simulink model "CM620A_MotAg0Meas"  (R2013b)
settings: Solver=FixedStepDiscrete  SolverMode=SingleTasking  StartTime=0.0  StopTime=1  FixedStep=0.0000625  RelTol=1e-3
undefined symbols (not defined in the file): ARCHGLBPRM_2PI_ULS_F32, COEFFTBLELMSIZE_CNT_U08, COEFFTBLSIZE_CNT_U08, CORRNTBLAGSTEPSIZE_MATRAD_F32, CORRNTBLSIDXOFFS_CNT_U16, CORRNTBLSIZE_CNT_U16, CORRNTBLSIZEMASK_CNT_U08, FLTINJ_MOTAG0MEAS_MOTCTRLMOTAG0MECL, FLTINJ_MOTAG0MEAS_TESTOK, MotAg0PrtclFlt, MOTAG0PRTCLFLTFAILSTEP_CNT_U16, MOTAG0PRTCLFLTPASSSTEP_CNT_U16, MOTAGDELTAPERCORRNPT_CNT_U16, MOTAGIDXMASK_CNT_U16, MotCtrlMotAg0ErrReg, NtcSts1, sigbuilder_block, SNSRAGMASK_CNT_U32, SNSRERRMASK_CNT_U32, SNSRERRNTCMASK_CNT_U08, SNSRVLTGFLTMASK_CNT_U32, SPIPARMASK_CNT_U32
libraries: simulink x28, FloatToFixd x1, NxtrMax x1, NxtrLim x1
(part 1 of 4)
settings Model: RequirementInfo="{}  %GIDa_ca294f38_ed7c_4fb9_8c54_f4d56271bfc7"  ModifiedHistory=Rev 008: Updated model to Matlab 2013B, added comments to show requirement linkage  Creator=nz3zln  LastModifiedBy=TZBSJD
settings SolverCC: AutoInsertRateTranBlk=on  InsertRTBMode=Always
settings DataIOCC: LimitDataPoints=off  SaveFormat=Structure  ReturnWorkspaceOutputs=on
settings OptimizationCC: BlockReduction=off  InlineParams=on  ZeroExternalMemoryAtStartup=off  ZeroInternalMemoryAtStartup=off  OptimizeModelRefInitCode=on  LifeSpan=1
settings DebuggingCC: SignalInfNanChecking=error  SignalRangeChecking=warning  UnderspecifiedInitializationDetection=Simplified  SolverPrmCheckMsg=error  InheritedTsInSrcMsg=error  DiscreteInheritContinuousMsg=error  SingleTaskRateTransMsg=error  TasksWithSamePriorityMsg=error  SigSpecEnsureSampleTimeMsg=error  CheckMatrixSingularityMsg=error  ParameterUnderflowMsg=error  ParameterPrecisionLossMsg=error  ParameterTunabilityLossMsg=error  FixptConstUnderflowMsg=warning  FixptConstOverflowMsg=warning  VectorMatrixConversionMsg=error  SignalLabelMismatchMsg=error  UnconnectedInputMsg=error  UnconnectedOutputMsg=error  UnconnectedLineMsg=error  SFcnCompatibilityMsg=error  UniqueDataStoreMsg=warning  BusObjectLabelMismatch=error  RootOutportRequireBusObject=error  AssertControl=DisableAll  ModelReferenceIOMsg=error  ModelReferenceVersionMismatchMessage=warning  ModelReferenceIOMismatchMessage=error  ModelReferenceCSMismatchMessage=warning  ModelReferenceDataLoggingMessage=error  StateNameClashWarn=warning  StrictBusMsg=ErrorOnBusTreatedAsVector  NonBusSignalsTreatedAsBus=error  SFUnexpectedBacktrackingDiag=error  SFInvalidInputDataAccessInChartInitDiag=error  SFNoUnconditionalDefaultTransitionDiag=error  SFTransitionOutsideNaturalParentDiag=error  SFUnconditionalTransitionShadowingDiag=error  SFUndirectedBroadcastEventsDiag=error
settings ModelReferenceCC: ModelReferenceNumInstancesAllowed=Single
settings RTWCC: SystemTargetFile=autosar.tlc  GenCodeOnly=on  TemplateMakefile=ert_default_tmf  Description=AUTOSAR  GenerateReport=on  ProcessScript=autosar_make_rtw_hook  LaunchReport=on
settings CodeAppCC: GenerateComments=off  IgnoreCustomStorageClasses=off  CustomSymbolStrType=$N$R$M  CustomSymbolStrBlkIO=$N$M  SimulinkBlockComments=off
settings STFCustomTargetCC: ParMdlRefBuildCompliant=on  CompOptLevelCompliant=on  IncludeMdlTerminateFcn=off  CombineOutputUpdateFcns=on  SuppressErrorStatus=on  ERTFirstTimeCompliant=on  ERTCustomFileBanners=on  SupportNonFinite=off  SupportComplex=off  SupportContinuousTime=off  SupportNonInlinedSFcns=off  MATLABClassNameForMDSCustomization=Simulink.SoftwareTarget.ERTCustomization  AutosarCompliant=on  GRTInterface=off  SystemTargetFile=autosar.tlc
settings ERTTargetCC: CodeReplacementLibrary=ANSI_C  ConcurrentExecutionCompliant=off  IncludeMdlTerminateFcn=off  SuppressErrorStatus=on  SupportNonFinite=off  SupportComplex=off  ModelStepFunctionPrototypeControlCompliant=off  CPPClassGenCompliant=off  AutosarCompliant=on  InlinedParameterPlacement=NonHierarchical  ERTCustomFileTemplate=example_file_process.tlc  EnableUserReplacementTypes=on

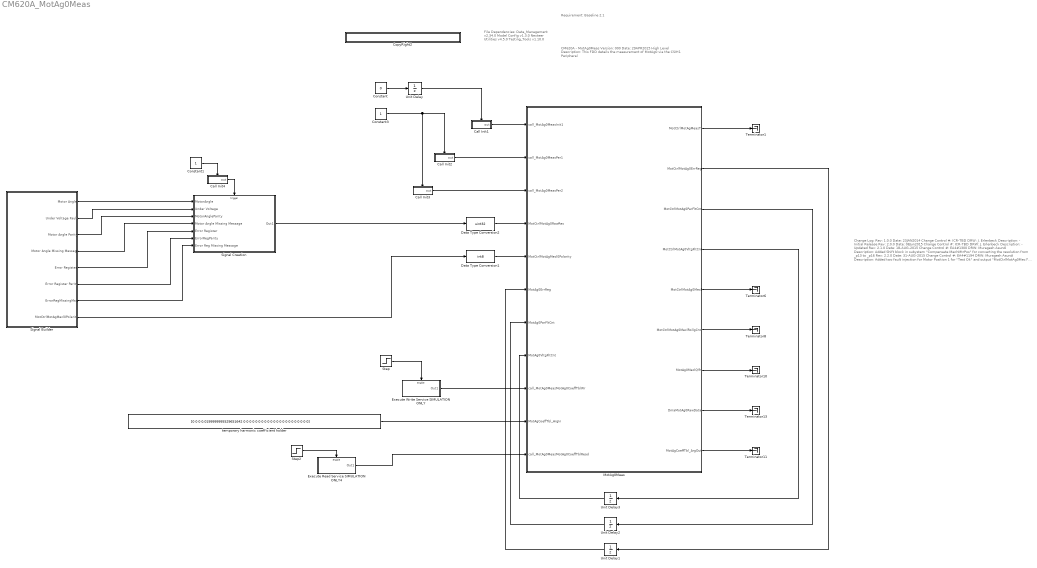
== system CM620A_MotAg0Meas ==
  note: CM620A - MotAg0Meas
      |
      | Version: 000
      | Date: 29APR2015
      |
      | High Level Description:
      | This FDD details the measurement of MotAg0 via the CSIH1 Peripheral
  note: Change Log:
      |
      | Rev: 1.0.0
      | Date: 23JAN2014
      | Change Control #: ICR-TBD
      | DRW: J. Erlenbeck
      | Description:
      | - Initial Release
      |
      | Rev: 2.0.0
      | Date: 08Jun2015
      | Change Control #: ICR-TBD
      | DRW: J. Erlenbeck
      | Description:
      | - Updated
      |
      | Rev: 2.1.0
      | Date: 18-AUG-2015
      | Change Control #: EA4#1300
      | DRW: Muragesh Asundi
      | Description: Added Shift block in subystem "Compensate MechMtrPos" for converting the resolution from _p13 to _p16
      |
      | Rev: 2.2.0
      | Date: 31-AUG-2015
      | Change Control #: EA4#1194
      | DRW: Muragesh Asundi
      | Description: Added two fault injection for Motor Position 1 for "Test Ok" and output "MotCtrlMotAg0Mecl"
      |
      | Rev: 2.3.0
      | Date: 09-SEP-2015
      | Change Control #: EA4#1404
      | DRW: J. Erlenbeck
      | Description: Updated for Anomaly fix to scaling
      |
      | Rev: 2.4.0
      | Date: 23-SEP-2015
      | Change Control #: EA4#1639
      | DRW: Muragesh Asundi
      | Description: Block "FltInj_u16" renamed to "FltInj_u0p16"
      |
      | Rev 3.0.0
      | Date - 30-Sep-2015
      | Change Control EA4#1725
      | DRW" Erlenbeck
      | Description: Changes to the Correction table process
      |
      | Rev 3.1.0
      | Date - 07-Oct-2015
      | Change Control EA4#1883
      | DRW" Erlenbeck
      | Description: Created routine in Init1 to initialize CSIH RAM to prevent ECC faults.  Place in some checks to to
      | verify denominator !=0 before division.
      |
      | Rev 3.2.0
      | Date - 18-Oct-2015
      | Change Control EA4#2085
      | DRW: Erlenbeck
      | Description: Removed routine in Init1 to initialize CSIH RAM to prevent ECC faults.  Changed some
      | typecasting in init function that prevented the function from running when NxtrMBDConfig.mat was run.
      | Replaced input signal creation from external file to one with signal builder.\
      |
      | Rev 3.2.1
      | Date - 18-Oct-2015
      | Change Control EA4#2085
      | DRW: Erlenbeck
      | Description: Minor changes needed for model to compile with NxtrMBDConfig.mat configuration.
      |
      | Rev 3.4.0
      | Date - 17-Dec-2015
      | Change Control EA4#3027
      | DRW: Erlenbeck
      | Description: Removed the read reset pointer.  Will be performed by the DMA.
      |
      | Rev 3.5.0
      | Date - 08-Mar-2016
      | Change Control EA4#3925, EA4#4645
      | DRW: Praveen(KPIT)
      | Description:
      | - M File change so that NVM MotAg0CoeffTbl.EngInit = []. Accordingly model updated to allign to this.
      | - As per anomaly CR EA4#3631, updated the variable MotCtrlMotAg0VltgFltCnt.WrittenIn field as MotAg1MeasPer1 in the .m file.
      |  -The maximum and minimum specified in the Data Type conversion block are removed and highlighted in the Model.
      |
      | Rev 3.6.0
      | Date - 07-Dec-2016
      | Change Control EA4#8812
      | DRW: Sai Desu
      | Description:
      | - Updated MotAg0VltgFltCnt.ReadIn in M-file from MotAg0MeasPer1 to MotAg0MeasPer2
  note: File Dependencies:
      | Data_Management v2.34.0
      | Model Config v1.3.0
      | Nexteer Utilities v4.5.0
      | Testing_Tools v1.10.0
  note: Requirement: Baseline 2.1
  Call Init1 : Subsystem  TreatAsAtomicUnit=on
  Call Init2 : Subsystem  TreatAsAtomicUnit=on
  Call Init3 : Subsystem  TreatAsAtomicUnit=on
  Call Init4 : Subsystem  TreatAsAtomicUnit=on
  Constant : Constant  Value=0  OutDataTypeStr=uint8
  Constant1 : Constant  OutDataTypeStr=int8
  Constant3 : Constant  OutDataTypeStr=int8
  CopyRight2 : Subsystem  Description=|  mask(Copyright Information){none=on}
      | Copyright info block.                                               
      |                                                                     
      | Place copyright information at the top of every subsystem in design.
      mask prompts: none "No parameters"
      mask help: Place copyright information at the top of every subsystem in design.
      mask Display:
      | NxtrConf = 'Nexteer Confidential';
      | 
      | sys = bdroot; %handle for the current model ("system")
      | first = get_param(sys,'Created');
      | first = first(end-3:end);  %year is last four digits
      | 
      | last = get_param(sys,'LastModifiedDate');
      | if isempty(last)
      |     last = datestr(now,'yyyy');
      | else
      |     last = last(end-3:end);
      | end
      | 
      | if strcmp(first,last)
      |     fprintf('%s -- Copyright %s Nexteer',NxtrConf,first)
      | else
      |     fprintf('%s -- %s%s- %s Nexteer',NxtrConf,char(169),first,last)
      | end
  Data Type Conversion1 : DataTypeConversion  OutDataTypeStr=int8
  Data Type Conversion2 : DataTypeConversion  OutDataTypeStr=uint32
  Execute Read Service SIMULATION ONLY4 : Subsystem  TreatAsAtomicUnit=on
  Execute Write Service SIMULATION ONLY : Subsystem  TreatAsAtomicUnit=on
  MotAg0Meas : Subsystem
  Signal Builder : Subsystem  Tag=STV Subsys  LoadFcn=sigbuilder_block('load');  StartFcn=sigbuilder_block('start');  StopFcn=sigbuilder_block('stop');  ClipboardFcn=sigbuilder_block('clipboard');  mask(Sigbuilder block){}
      mask help: Simulink:masks:SigbuilderBlock_MD
      mask init:
      | if ~strcmp(get_param(bdroot(gcbh),'SimulationStatus'),'stopped') tuvar = sigbuilder_block('maskInit'); end
      settings: CopyFcn=sigbuilder_block('copy');  DeleteFcn=sigbuilder_block('delete');  ModelCloseFcn=sigbuilder_block('modelClose');  PreSaveFcn=sigbuilder_block('preSave');  PauseFcn=sigbuilder_block('pause');  ContinueFcn=sigbuilder_block('continue');  NameChangeFcn=sigbuilder_block('namechange');  OpenFcn=sigbuilder_block('open',[306 215.379 548.69 396.621 ]);  CloseFcn=sigbuilder_block('close');
      mask Display: plot(0, 0, 100, 100,[2, 2, 32, 32, 2], [68, 8, 8, 68, 68],[32, 2], [38, 38], [32, 19, 2],[53, 60, 44], [32, 17, 17, 2],[16, 16, 31, 31]);txt = getActiveGroup(gcbh);text(2, 100, txt,'verticalAlignment', 'top');
  Signal Creation : Subsystem
  Step : Step  Time=0.05  SampleTime=0
  Step2 : Step  Time=0.8  SampleTime=0
  Terminator{1,6,8,10..11,13} (6 alike) : Terminator
  Unit Delay : UnitDelay  InitialCondition=1  SampleTime=-1
  Unit Delay1 : UnitDelay  SampleTime=-1
  Unit Delay2 : UnitDelay  SampleTime=-1
  Unit Delay3 : UnitDelay  SampleTime=-1
  temporary harmonic coefficient holder : Constant  Value=[0 0 0 0.0199999995529651642 0 0 0 0 0 0 0 0 0 0 0 0 0 0 0 0 0 0 0 0 0 0]  OutDataTypeStr=single
  wires:
  Constant/1 -> Unit Delay/1
  Unit Delay/1 -> Call Init1/Enable
  Constant3/1 -> Call Init2/Enable, Call Init3/Enable
  Call Init1/1(out) -> MotAg0Meas/1(call_MotAg0MeasInit1)
  Call Init2/1(out) -> MotAg0Meas/2(call_MotAg0MeasPer1)
  Signal Creation/1(Out1) -> Data Type Conversion2/1
  Data Type Conversion2/1 -> MotAg0Meas/4(MotCtrlMotAg0RawRes)
  Call Init3/1(out) -> MotAg0Meas/3(call_MotAg0MeasPer2)
  Step/1 -> Execute Write Service SIMULATION ONLY/Enable
  Execute Write Service SIMULATION ONLY/1(Out1) -> MotAg0Meas/9(call_MotAg0MeasMotAg0CoeffTblWr)
  MotAg0Meas/1(MotCtrlMotAgMeasTi) -> Terminator1/1
  MotAg0Meas/5(MotCtrlMotAg0Mecl) -> Terminator6/1
  MotAg0Meas/6(MotCtrlMotAg0MeclRollgCntr) -> Terminator8/1
  MotAg0Meas/7(MotAg0MeclQlfr) -> Terminator10/1
  MotAg0Meas/8(DmaMotAg0RawData) -> Terminator13/1
  Step2/1 -> Execute Read Service SIMULATION ONLY4/Enable
  Execute Read Service SIMULATION ONLY4/1(Out1) -> MotAg0Meas/11(call_MotAg0MeasMotAg0CoeffTblRead)
  temporary harmonic coefficient holder/1 -> MotAg0Meas/10(MotAgCoeffTbl_ArgIn)
  MotAg0Meas/9(MotAgCoeffTbl_ArgOut) -> Terminator11/1
  MotAg0Meas/2(MotCtrlMotAg0ErrReg) -> Unit Delay1/1
  Unit Delay1/1 -> MotAg0Meas/6(MotAg0ErrReg)
  MotAg0Meas/3(MotCtrlMotAg0ParFltCnt) -> Unit Delay2/1
  Unit Delay2/1 -> MotAg0Meas/7(MotAg0ParFltCnt)
  MotAg0Meas/4(MotCtrlMotAg0VltgFltCnt) -> Unit Delay3/1
  Unit Delay3/1 -> MotAg0Meas/8(MotAg0VltgFltCnt)
  Constant1/1 -> Call Init4/Enable
  Call Init4/1(out) -> Signal Creation/Trigger
  Signal Builder/1(Motor Angle) -> Signal Creation/1(MotorAngle)
  Signal Builder/2(Under Voltage Fault) -> Signal Creation/2(Under Voltage)
  Signal Builder/3(Motor Angle Parity) -> Signal Creation/3(MotorAngleParity)
  Signal Builder/5(Error Register) -> Signal Creation/5(Error Register)
  Signal Builder/6(Error Register Parity) -> Signal Creation/6(ErrorRegParity)
  Signal Builder/8(MotCtrlMotAgMecl0Polarity) -> Data Type Conversion1/1
  Data Type Conversion1/1 -> MotAg0Meas/5(MotCtrlMotAgMecl0Polarity)
  Signal Builder/4(Motor Angle Missing Message) -> Signal Creation/4(Motor Angle Missing Message)
  Signal Builder/7(ErrorRegMissingMsg) -> Signal Creation/7(Error Reg Missing Message)

== system CM620A_MotAg0Meas/Call Init1 ==
  Enable : EnablePort
  Function Call Trigger : simulink/Ports & Subsystems/Function-Call Generator  RequirementInfo={} %GIDa_ff755a2e_49d1_45f7_8591_3ce0ef475338  sample_time=0.002  numberOfIterations=1
  out : Outport
  wires:
  Function Call Trigger/1 -> out/1

== system CM620A_MotAg0Meas/Call Init2 ==
  Enable : EnablePort
  Function Call Trigger : simulink/Ports & Subsystems/Function-Call Generator  RequirementInfo={} %GIDa_6dd05ab1_f91b_4d7a_a0ec_1170d213fa7b  sample_time=0.0005  numberOfIterations=1
  out : Outport
  wires:
  Function Call Trigger/1 -> out/1

== system CM620A_MotAg0Meas/Call Init3 ==
  Enable : EnablePort
  Function Call Trigger : simulink/Ports & Subsystems/Function-Call Generator  RequirementInfo={} %GIDa_9bd65ccd_39f3_4e48_9d09_4984d13bbcbb  sample_time=0.002  numberOfIterations=1
  out : Outport
  wires:
  Function Call Trigger/1 -> out/1

== system CM620A_MotAg0Meas/Call Init4 ==
  Enable : EnablePort
  Function Call Trigger : simulink/Ports & Subsystems/Function-Call Generator  RequirementInfo={} %GIDa_6dd05ab1_f91b_4d7a_a0ec_1170d213fa7b  sample_time=0.0005  numberOfIterations=1
  out : Outport
  wires:
  Function Call Trigger/1 -> out/1

== system CM620A_MotAg0Meas/CopyRight2 ==

== system CM620A_MotAg0Meas/Execute Read Service SIMULATION ONLY4 ==
  Enable : EnablePort
  Function-Call Generator1 : simulink/Ports & Subsystems/Function-Call Generator  sample_time=0.0000625  numberOfIterations=1
  Out1 : Outport
  wires:
  Function-Call Generator1/1 -> Out1/1

== system CM620A_MotAg0Meas/Execute Write Service SIMULATION ONLY ==
  Enable : EnablePort
  Function-Call Generator1 : simulink/Ports & Subsystems/Function-Call Generator  sample_time=0.0000625  numberOfIterations=1
  Out1 : Outport
  wires:
  Function-Call Generator1/1 -> Out1/1

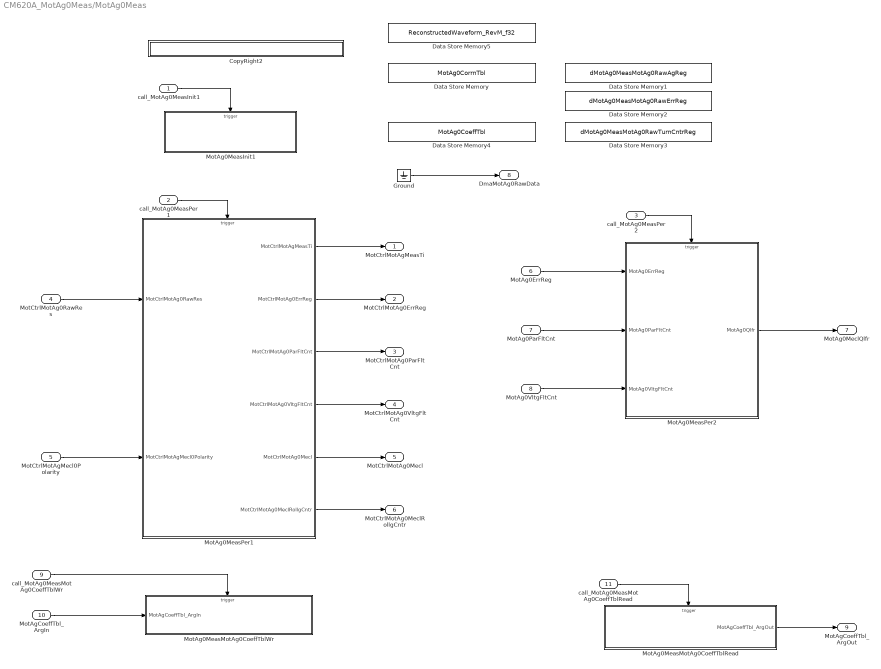
== system CM620A_MotAg0Meas/MotAg0Meas ==
  call_MotAg0MeasInit1 : Inport  RequirementInfo={} %GIDa_18b4b7a7_d8ff_42fd_afd9_8fbc558fb7ae
  call_MotAg0MeasPer1 : Inport  RequirementInfo={} %GIDa_8c56c68f_1996_47ee_bda4_35b4dc112bcf  Port=2
  call_MotAg0MeasPer2 : Inport  RequirementInfo={} %GIDa_7b28921c_189e_46dc_b03b_f7509365a7f9  Port=3
  MotCtrlMotAg0RawRes : Inport  RequirementInfo={'linktype_rmi_doors' '0000c47b (/ESG Group/FDD Module Requirements/EA4 Specific/CM620A_MotAg0Meas)' '#CM620A_48' 'true' 'REQ: CM620A_48' '' } %GIDa_768985a4_e900_425c_ae1d_47338650e664  Port=4
  MotCtrlMotAgMecl0Polarity : Inport  RequirementInfo={'linktype_rmi_doors' '0000c47b (/ESG Group/FDD Module Requirements/EA4 Specific/CM620A_MotAg0Meas)' '#CM620A_49' 'true' 'REQ: CM620A_49' '' } %GIDa_8ed9d5d5_f39e_4ce8_8e17_7324d3fb8e4d  Port=5  OutDataTypeStr=int8
  MotAg0ErrReg : Inport  Port=6
  MotAg0ParFltCnt : Inport  Port=7
  MotAg0VltgFltCnt : Inport  Port=8
  call_MotAg0MeasMotAg0CoeffTblWr : Inport  Port=9
  MotAgCoeffTbl_ArgIn : Inport  Port=10
  call_MotAg0MeasMotAg0CoeffTblRead : Inport  Port=11
  CopyRight2 : Subsystem  Description=|  mask(Copyright Information){none=on}
      | Copyright info block.                                               
      |                                                                     
      | Place copyright information at the top of every subsystem in design.
      mask prompts: none "No parameters"
      mask help: Place copyright information at the top of every subsystem in design.
      mask Display:
      | NxtrConf = 'Nexteer Confidential';
      | 
      | sys = bdroot; %handle for the current model ("system")
      | first = get_param(sys,'Created');
      | first = first(end-3:end);  %year is last four digits
      | 
      | last = get_param(sys,'LastModifiedDate');
      | if isempty(last)
      |     last = datestr(now,'yyyy');
      | else
      |     last = last(end-3:end);
      | end
      | 
      | if strcmp(first,last)
      |     fprintf('%s -- Copyright %s Nexteer',NxtrConf,first)
      | else
      |     fprintf('%s -- %s%s- %s Nexteer',NxtrConf,char(169),first,last)
      | end
  Data Store Memory : DataStoreMemory  DataStoreName=MotAg0CorrnTbl  InitialValue=[]  StateMustResolveToSignalObject=on
  Data Store Memory1 : DataStoreMemory  DataStoreName=dMotAg0MeasMotAg0RawAgReg  OutDataTypeStr=uint32  StateMustResolveToSignalObject=on
  Data Store Memory2 : DataStoreMemory  DataStoreName=dMotAg0MeasMotAg0RawErrReg  OutDataTypeStr=uint32
  Data Store Memory3 : DataStoreMemory  DataStoreName=dMotAg0MeasMotAg0RawTurnCntrReg  OutDataTypeStr=uint32
  Data Store Memory4 : DataStoreMemory  DataStoreName=MotAg0CoeffTbl  InitialValue=[]  StateMustResolveToSignalObject=on
  Data Store Memory5 : DataStoreMemory  DataStoreName=ReconstructedWaveform_RevM_f32  InitialValue=zeros(128,1)  OutDataTypeStr=single
  Ground : Ground
  MotAg0MeasInit1 : Subsystem
  MotAg0MeasMotAg0CoeffTblRead : Subsystem  RequirementInfo="{'linktype_rmi_doors' '0000c47b (/ESG Group/FDD Module Requirements/EA4 Specific/CM620A_MotAg0Meas)' '#CM620A_104' 'true' 'REQ:  CM620A_104' '' } %GIDa_efd3f6e0_f9ec_43d5_8495_6ebd7018f9f2"
  MotAg0MeasMotAg0CoeffTblWr : Subsystem  RequirementInfo={'linktype_rmi_doors' '0000c47b (/ESG Group/FDD Module Requirements/EA4 Specific/CM620A_MotAg0Meas)' '#CM620A_32' 'true' 'REQ: CM620A_32' '' } %GIDa_58c26980_fa56_4411_8dac_1a94429c65df
  MotAg0MeasPer1 : Subsystem  TreatAsAtomicUnit=on
  MotAg0MeasPer2 : Subsystem  TreatAsAtomicUnit=on
  MotCtrlMotAgMeasTi : Outport  RequirementInfo={'linktype_rmi_doors' '0000c47b (/ESG Group/FDD Module Requirements/EA4 Specific/CM620A_MotAg0Meas)' '#CM620A_67' 'true' 'REQ: CM620A_67' '' } %GIDa_db4c44ad_deed_47c2_80de_3c33b65dc64c
  MotCtrlMotAg0ErrReg : Outport  Port=2
  MotCtrlMotAg0ParFltCnt : Outport  Port=3
  MotCtrlMotAg0VltgFltCnt : Outport  Port=4
  MotCtrlMotAg0Mecl : Outport  RequirementInfo={'linktype_rmi_doors' '0000c47b (/ESG Group/FDD Module Requirements/EA4 Specific/CM620A_MotAg0Meas)' '#CM620A_66' 'true' 'REQ: CM620A_66' '' } %GIDa_a40ef296_4e6e_4397_997e_05fcb9e70ed5  Port=5
  MotCtrlMotAg0MeclRollgCntr : Outport  Port=6
  MotAg0MeclQlfr : Outport  RequirementInfo={'linktype_rmi_doors' '0000c47b (/ESG Group/FDD Module Requirements/EA4 Specific/CM620A_MotAg0Meas)' '#CM620A_105' 'true' 'REQ: CM620A_105' '' } %GIDa_eb095ceb_60c6_4658_947c_a9047682a36a  Port=7
  DmaMotAg0RawData : Outport  Port=8
  MotAgCoeffTbl_ArgOut : Outport  Port=9
  wires:
  MotCtrlMotAgMecl0Polarity/1 -> MotAg0MeasPer1/2(MotCtrlMotAgMecl0Polarity)
  call_MotAg0MeasInit1/1 -> MotAg0MeasInit1/Trigger
  call_MotAg0MeasPer1/1 -> MotAg0MeasPer1/Trigger
  MotCtrlMotAg0RawRes/1 -> MotAg0MeasPer1/1(MotCtrlMotAg0RawRes)
  MotAg0MeasPer1/1(MotCtrlMotAgMeasTi) -> MotCtrlMotAgMeasTi/1
  MotAg0MeasPer1/2(MotCtrlMotAg0ErrReg) -> MotCtrlMotAg0ErrReg/1
  MotAg0MeasPer1/4(MotCtrlMotAg0VltgFltCnt) -> MotCtrlMotAg0VltgFltCnt/1
  MotAg0MeasPer1/3(MotCtrlMotAg0ParFltCnt) -> MotCtrlMotAg0ParFltCnt/1
  MotAg0MeasPer1/6(MotCtrlMotAg0MeclRollgCntr) -> MotCtrlMotAg0MeclRollgCntr/1
  call_MotAg0MeasPer2/1 -> MotAg0MeasPer2/Trigger
  MotAg0MeasPer2/1(MotAg0Qlfr) -> MotAg0MeclQlfr/1
  call_MotAg0MeasMotAg0CoeffTblWr/1 -> MotAg0MeasMotAg0CoeffTblWr/Trigger
  Ground/1 -> DmaMotAg0RawData/1
  MotAgCoeffTbl_ArgIn/1 -> MotAg0MeasMotAg0CoeffTblWr/1(MotAgCoeffTbl_ArgIn)
  call_MotAg0MeasMotAg0CoeffTblRead/1 -> MotAg0MeasMotAg0CoeffTblRead/Trigger
  MotAg0MeasPer1/5(MotCtrlMotAg0Mecl) -> MotCtrlMotAg0Mecl/1
  MotAg0MeasMotAg0CoeffTblRead/1(MotAgCoeffTbl_ArgOut) -> MotAgCoeffTbl_ArgOut/1
  MotAg0ErrReg/1 -> MotAg0MeasPer2/1(MotAg0ErrReg)
  MotAg0ParFltCnt/1 -> MotAg0MeasPer2/2(MotAg0ParFltCnt)
  MotAg0VltgFltCnt/1 -> MotAg0MeasPer2/3(MotAg0VltgFltCnt)

== system CM620A_MotAg0Meas/Signal Builder ==
  Demux : Demux  Tag=STV Demux  Outputs=8
  FromWs : FromWorkspace  Tag=STV FromWs  VariableName=tuvar  SampleTime=0
      SigBuilderData=|
      | common.afterFinalStr = 'Extrapolate'
      | common.sampleTime = 0
      | dataSet.timeRange = [0 2]
      | dataSet.name = 'Group 1'
      | sbobj.Groups.Name = 'Group 1'
      | sbobj.Groups.Signals(1).Name = 'Motor Angle'
      | sbobj.Groups.Signals(1).XData = [0 1 2]
      | sbobj.Groups.Signals(1).YData = [0 1500 -900]
      | sbobj.Groups.Signals(2).Name = 'Under Voltage Fault'
      | sbobj.Groups.Signals(2).XData = [0 0.288 0.288 0.326 0.326 2]
      | sbobj.Groups.Signals(2).YData = [0 0 1 1 0 0]
      | sbobj.Groups.Signals(3).Name = 'Motor Angle Parity'
      | sbobj.Groups.Signals(3).XData = [0 0.201 0.201 0.21 0.21 2]
      | sbobj.Groups.Signals(3).YData = [0 0 1 1 0 0]
      | sbobj.Groups.Signals(4).Name = 'Motor Angle Missing Message'
      | sbobj.Groups.Signals(4).XData = [0 0.534 0.534 0.544 0.544 2]
      | sbobj.Groups.Signals(4).YData = [0 0 1 1 0 0]
      | sbobj.Groups.Signals(5).Name = 'Error Register'
      | sbobj.Groups.Signals(5).XData = [0 0.864 0.864 0.898 0.898 0.962 0.962 1.056 1.056 1.144 1.144 1.2 1.2 1.264 1.264 2]
      | sbobj.Groups.Signals(5).YData = [0 0 1 1 2 2 4 4 0 0 8 8 6 6 0 0]
      | sbobj.Groups.Signals(6).Name = 'Error Register Parity'
      | sbobj.Groups.Signals(6).XData = [0 2]
      | sbobj.Groups.Signals(6).YData = [0 0]
      | sbobj.Groups.Signals(7).Name = 'ErrorRegMissingMsg'
      | sbobj.Groups.Signals(7).XData = [0 1.608 1.608 1.632 1.632 2]
      | sbobj.Groups.Signals(7).YData = [0 0 1 1 0 0]
      | sbobj.Groups.Signals(8).Name = 'MotCtrlMotAgMecl0Polarity'
      | sbobj.Groups.Signals(8).XData = [0 1.792 1.792 2]
      | sbobj.Groups.Signals(8).YData = [1 1 -1 -1]
      | sbobj.Groups.TimeRange = [0 2]
  Motor Angle : Outport  Tag=STV Outport
  Under Voltage Fault : Outport  Tag=STV Outport  Port=2
  Motor Angle Parity : Outport  Tag=STV Outport  Port=3
  Motor Angle Missing Message : Outport  Tag=STV Outport  Port=4
  Error Register : Outport  Tag=STV Outport  Port=5
  Error Register Parity : Outport  Tag=STV Outport  Port=6
  ErrorRegMissingMsg : Outport  Tag=STV Outport  Port=7
  MotCtrlMotAgMecl0Polarity : Outport  Tag=STV Outport  Port=8
  wires:
  FromWs/1 -> Demux/1
  Demux/1 -> Motor Angle/1
  Demux/2 -> Under Voltage Fault/1
  Demux/3 -> Motor Angle Parity/1
  Demux/4 -> Motor Angle Missing Message/1
  Demux/5 -> Error Register/1
  Demux/6 -> Error Register Parity/1
  Demux/7 -> ErrorRegMissingMsg/1
  Demux/8 -> MotCtrlMotAgMecl0Polarity/1

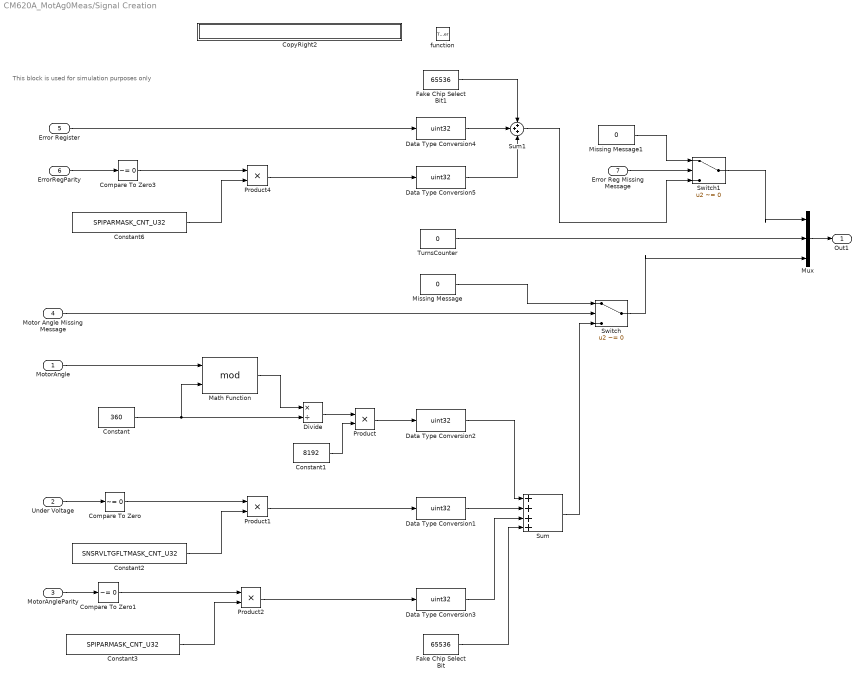
== system CM620A_MotAg0Meas/Signal Creation ==
  note: This block is used for simulation purposes only
  MotorAngle : Inport  RequirementInfo={} %GIDa_6ba4f99d_d8c8_4d56_8de2_9aa660055d1e
  Under Voltage : Inport  RequirementInfo={} %GIDa_53ff4c03_a3ae_416f_9367_d7418c7aacfd  Port=2
  MotorAngleParity : Inport  RequirementInfo={} %GIDa_86b900b1_8486_4794_8269_b5193284bc43  Port=3
  Motor Angle Missing Message : Inport  RequirementInfo={} %GIDa_e94cbc20_207e_45b6_8ada_f333992826fd  Port=4
  Error Register : Inport  RequirementInfo={} %GIDa_3b8fba3c_7125_490c_a301_802e8993f682  Port=5
  ErrorRegParity : Inport  RequirementInfo={} %GIDa_46ffa422_a9f2_4bcd_a096_e28769753b36  Port=6
  Error Reg Missing Message : Inport  RequirementInfo={} %GIDa_bd8e49e0_ef4b_4ada_acdb_75191b229f13  Port=7
  function : TriggerPort  TriggerType=function-call
  Compare To Zero : simulink/Logic and Bit Operations/Compare To Zero  relop=~=  OutDataTypeStr=uint8
  Compare To Zero1 : simulink/Logic and Bit Operations/Compare To Zero  relop=~=  OutDataTypeStr=uint8
  Compare To Zero3 : simulink/Logic and Bit Operations/Compare To Zero  relop=~=  OutDataTypeStr=uint8
  Constant : Constant  Value=360
  Constant1 : Constant  Value=8192
  Constant2 : Constant  Value=SNSRVLTGFLTMASK_CNT_U32
  Constant3 : Constant  Value=SPIPARMASK_CNT_U32
  Constant6 : Constant  Value=SPIPARMASK_CNT_U32
  CopyRight2 : Subsystem  Description=|  mask(Copyright Information){none=on}
      | Copyright info block.                                               
      |                                                                     
      | Place copyright information at the top of every subsystem in design.
      mask prompts: none "No parameters"
      mask help: Place copyright information at the top of every subsystem in design.
      mask Display:
      | NxtrConf = 'Nexteer Confidential';
      | 
      | sys = bdroot; %handle for the current model ("system")
      | first = get_param(sys,'Created');
      | first = first(end-3:end);  %year is last four digits
      | 
      | last = get_param(sys,'LastModifiedDate');
      | if isempty(last)
      |     last = datestr(now,'yyyy');
      | else
      |     last = last(end-3:end);
      | end
      | 
      | if strcmp(first,last)
      |     fprintf('%s -- Copyright %s Nexteer',NxtrConf,first)
      | else
      |     fprintf('%s -- %s%s- %s Nexteer',NxtrConf,char(169),first,last)
      | end
  Data Type Conversion{1..5} (5 alike) : DataTypeConversion  OutDataTypeStr=uint32
  Divide : Product  Inputs=*/
  Fake Chip Select Bit : Constant  Value=65536  OutDataTypeStr=uint32
  Fake Chip Select Bit1 : Constant  Value=65536  OutDataTypeStr=uint32
  Math Function : Math  Operator=mod  SaturateOnIntegerOverflow=on
  Missing Message : Constant  Value=0  OutDataTypeStr=uint32
  Missing Message1 : Constant  Value=0  OutDataTypeStr=uint32
  Mux : Mux  Inputs=3
  Product{,1..2,4} (4 alike) : Product
  Sum : Sum  Inputs=++++
  Sum1 : Sum  Inputs=+++
  Switch : Switch  Criteria=u2 ~= 0
  Switch1 : Switch  Criteria=u2 ~= 0
  TurnsCounter : Constant  Value=0  OutDataTypeStr=uint32
  Out1 : Outport
  wires:
  MotorAngle/1 -> Math Function/1
  Constant/1 -> Math Function/2, Divide/2
  Math Function/1 -> Divide/1
  Divide/1 -> Product/1
  Constant1/1 -> Product/2
  Product/1 -> Data Type Conversion2/1
  Mux/1 -> Out1/1
  Under Voltage/1 -> Compare To Zero/1
  Compare To Zero/1 -> Product1/1
  Constant2/1 -> Product1/2
  MotorAngleParity/1 -> Compare To Zero1/1
  Compare To Zero1/1 -> Product2/1
  Constant3/1 -> Product2/2
  Data Type Conversion2/1 -> Sum/1
  Product1/1 -> Data Type Conversion1/1
  Product2/1 -> Data Type Conversion3/1
  Data Type Conversion1/1 -> Sum/2
  Data Type Conversion3/1 -> Sum/3
  TurnsCounter/1 -> Mux/2
  ErrorRegParity/1 -> Compare To Zero3/1
  Compare To Zero3/1 -> Product4/1
  Constant6/1 -> Product4/2
  Product4/1 -> Data Type Conversion5/1
  Sum1/1 -> Switch1/3
  Error Register/1 -> Data Type Conversion4/1
  Fake Chip Select Bit/1 -> Sum/4
  Motor Angle Missing Message/1 -> Switch/2
  Missing Message/1 -> Switch/1
  Sum/1 -> Switch/3
  Switch/1 -> Mux/3
  Missing Message1/1 -> Switch1/1
  Error Reg Missing Message/1 -> Switch1/2
  Switch1/1 -> Mux/1
  Fake Chip Select Bit1/1 -> Sum1/1
  Data Type Conversion4/1 -> Sum1/2
  Data Type Conversion5/1 -> Sum1/3

== system CM620A_MotAg0Meas/MotAg0Meas/CopyRight2 ==

== system CM620A_MotAg0Meas/MotAg0Meas/MotAg0MeasInit1 ==
  function : TriggerPort  TriggerType=function-call
  Compute Correction Table : Subsystem  Priority=30  TreatAsAtomicUnit=on
      settings: AttributesFormatString=|
      | Priority:
      | %<Priority>
  CopyRight2 : Subsystem  Description=|  mask(Copyright Information){none=on}
      | Copyright info block.                                               
      |                                                                     
      | Place copyright information at the top of every subsystem in design.
      mask prompts: none "No parameters"
      mask help: Place copyright information at the top of every subsystem in design.
      mask Display:
      | NxtrConf = 'Nexteer Confidential';
      | 
      | sys = bdroot; %handle for the current model ("system")
      | first = get_param(sys,'Created');
      | first = first(end-3:end);  %year is last four digits
      | 
      | last = get_param(sys,'LastModifiedDate');
      | if isempty(last)
      |     last = datestr(now,'yyyy');
      | else
      |     last = last(end-3:end);
      | end
      | 
      | if strcmp(first,last)
      |     fprintf('%s -- Copyright %s Nexteer',NxtrConf,first)
      | else
      |     fprintf('%s -- %s%s- %s Nexteer',NxtrConf,char(169),first,last)
      | end
  Initialize CSIH Registers : Subsystem  Priority=20  TreatAsAtomicUnit=on
      settings: AttributesFormatString=|
      | Priority:
      | %<Priority>

== system CM620A_MotAg0Meas/MotAg0Meas/MotAg0MeasMotAg0CoeffTblRead ==
  Trigger : TriggerPort  TriggerType=function-call  PortDimensions=1
  Copyright1 : Subsystem  Description=|  mask(Copyright Information){none=on}
      | Copyright info block.                                               
      |                                                                     
      | Place copyright information at the top of every subsystem in design.
      mask prompts: none "No parameters"
      mask help: Place copyright information at the top of every subsystem in design.
      mask Display:
      | NxtrConf = 'Nexteer Confidential';
      | 
      | sys = bdroot; %handle for the current model ("system")
      | first = get_param(sys,'Created');
      | if(isempty(first))
      |     first = datestr(now,'yyyy');
      | else
      |     first = first(end-3:end);  %year is last four digits
      | end
      | 
      | last = get_param(sys,'LastModifiedDate');
      | if isempty(last)
      |     last = datestr(now,'yyyy');
      | else
      |     last = last(end-3:end);
      | end
      | 
      | if strcmp(first,last)
      |     fprintf('%s\nCopyright  %s Nexteer',NxtrConf,first);
      | else
      |     fprintf('%s\n%s%s-%s Nexteer',NxtrConf,char(169),first,last);
      | end
  Data Store Read : DataStoreRead  DataStoreName=MotAg0CoeffTbl
  MotAgCoeffTbl_ArgOut : Outport
  wires:
  Data Store Read/1 -> MotAgCoeffTbl_ArgOut/1

== system CM620A_MotAg0Meas/MotAg0Meas/MotAg0MeasMotAg0CoeffTblWr ==
  MotAgCoeffTbl_ArgIn : Inport
  Trigger : TriggerPort  TriggerType=function-call  PortDimensions=1
  Block Changed = True : Constant  OutDataTypeStr=boolean
  Copyright1 : Subsystem  Description=|  mask(Copyright Information){none=on}
      | Copyright info block.                                               
      |                                                                     
      | Place copyright information at the top of every subsystem in design.
      mask prompts: none "No parameters"
      mask help: Place copyright information at the top of every subsystem in design.
      mask Display:
      | NxtrConf = 'Nexteer Confidential';
      | 
      | sys = bdroot; %handle for the current model ("system")
      | first = get_param(sys,'Created');
      | if(isempty(first))
      |     first = datestr(now,'yyyy');
      | else
      |     first = first(end-3:end);  %year is last four digits
      | end
      | 
      | last = get_param(sys,'LastModifiedDate');
      | if isempty(last)
      |     last = datestr(now,'yyyy');
      | else
      |     last = last(end-3:end);
      | end
      | 
      | if strcmp(first,last)
      |     fprintf('%s\nCopyright  %s Nexteer',NxtrConf,first);
      | else
      |     fprintf('%s\n%s%s-%s Nexteer',NxtrConf,char(169),first,last);
      | end
  Data Store Write : DataStoreWrite  DataStoreName=MotAg0CoeffTbl
  MotAg0CoeffTbl_SetRamBlockStatus : Subsystem
  wires:
  Block Changed = True/1 -> MotAg0CoeffTbl_SetRamBlockStatus/1(BlockChanged)
  MotAgCoeffTbl_ArgIn/1 -> Data Store Write/1

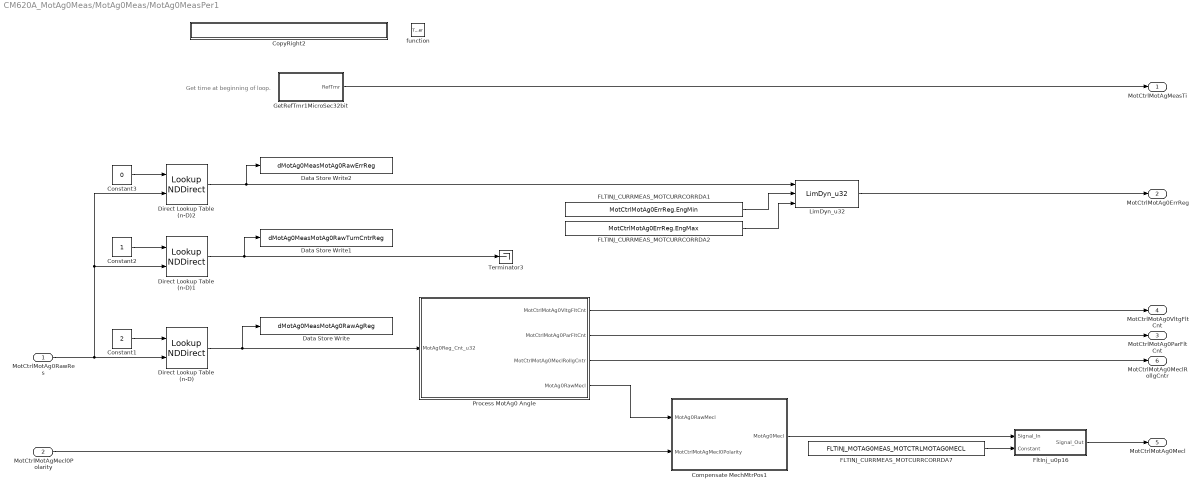
== system CM620A_MotAg0Meas/MotAg0Meas/MotAg0MeasPer1 ==
  note: Get time at beginning of loop.
  MotCtrlMotAg0RawRes : Inport
  MotCtrlMotAgMecl0Polarity : Inport  Port=2
  function : TriggerPort  TriggerType=function-call
  Compensate MechMtrPos1 : Subsystem  RequirementInfo="{'linktype_rmi_doors' '0000c47b (/ESG Group/FDD Module Requirements/EA4 Specific/CM620A_MotAg0Meas)' '#CM620A_118' 'true' 'REQ:  CM620A_118' '' } %GIDa_7e1af811_171e_4f01_9746_2e074d70b9e9"
  Constant1 : Constant  Value=2
  Constant2 : Constant
  Constant3 : Constant  Value=0
  CopyRight2 : Subsystem  Description=|  mask(Copyright Information){none=on}
      | Copyright info block.                                               
      |                                                                     
      | Place copyright information at the top of every subsystem in design.
      mask prompts: none "No parameters"
      mask help: Place copyright information at the top of every subsystem in design.
      mask Display:
      | NxtrConf = 'Nexteer Confidential';
      | 
      | sys = bdroot; %handle for the current model ("system")
      | first = get_param(sys,'Created');
      | first = first(end-3:end);  %year is last four digits
      | 
      | last = get_param(sys,'LastModifiedDate');
      | if isempty(last)
      |     last = datestr(now,'yyyy');
      | else
      |     last = last(end-3:end);
      | end
      | 
      | if strcmp(first,last)
      |     fprintf('%s -- Copyright %s Nexteer',NxtrConf,first)
      | else
      |     fprintf('%s -- %s%s- %s Nexteer',NxtrConf,char(169),first,last)
      | end
  Data Store Write : DataStoreWrite  DataStoreName=dMotAg0MeasMotAg0RawAgReg
  Data Store Write1 : DataStoreWrite  DataStoreName=dMotAg0MeasMotAg0RawTurnCntrReg
  Data Store Write2 : DataStoreWrite  DataStoreName=dMotAg0MeasMotAg0RawErrReg
  Direct Lookup Table (n-D) : LookupNDDirect  NumberOfTableDimensions=1  TableIsInput=on
  Direct Lookup Table (n-D)1 : LookupNDDirect  NumberOfTableDimensions=1  TableIsInput=on
  Direct Lookup Table (n-D)2 : LookupNDDirect  NumberOfTableDimensions=1  TableIsInput=on
  FLTINJ_CURRMEAS_MOTCURRCORRDA1 : Constant  Value=MotCtrlMotAg0ErrReg.EngMin  OutDataTypeStr=uint32
  FLTINJ_CURRMEAS_MOTCURRCORRDA2 : Constant  Value=MotCtrlMotAg0ErrReg.EngMax  OutDataTypeStr=uint32
  FLTINJ_CURRMEAS_MOTCURRCORRDA7 : Constant  Value=FLTINJ_MOTAG0MEAS_MOTCTRLMOTAG0MECL
  FltInj_u0p16 : Subsystem  RequirementInfo={'linktype_rmi_doors' '0000c47b (/ESG Group/FDD Module Requirements/EA4 Specific/CM620A_MotAg0Meas)' '#CM620A_112' 'true' 'REQ: CM620A_112' '' } %GIDa_3bef8a1b_02a8_416a_94d4_ebb87c2c8610  TreatAsAtomicUnit=on  VariantControl=FltInj_sim  mask(Fault_Injection){}
      mask help: Fault Injection is a simulation only block for EA3 programs.
  GetRefTmr1MicroSec32bit : Subsystem  Priority=1  TreatAsAtomicUnit=on
      settings: AttributesFormatString=|
      | Priority:
      | %<Priority>
  LimDyn_u32 : NxtrLim/LimDyn_u32
  Process MotAg0 Angle : Subsystem
  Terminator3 : Terminator
  MotCtrlMotAgMeasTi : Outport
  MotCtrlMotAg0ErrReg : Outport  Port=2
  MotCtrlMotAg0ParFltCnt : Outport  Port=3
  MotCtrlMotAg0VltgFltCnt : Outport  Port=4
  MotCtrlMotAg0Mecl : Outport  Port=5
  MotCtrlMotAg0MeclRollgCntr : Outport  Port=6
  wires:
  GetRefTmr1MicroSec32bit/1(RefTmr) -> MotCtrlMotAgMeasTi/1
  Constant1/1 -> Direct Lookup Table (n-D)/1
  MotCtrlMotAg0RawRes/1 -> Direct Lookup Table (n-D)2/2, Direct Lookup Table (n-D)1/2, Direct Lookup Table (n-D)/2
  Constant2/1 -> Direct Lookup Table (n-D)1/1
  Constant3/1 -> Direct Lookup Table (n-D)2/1
  Process MotAg0 Angle/1(MotCtrlMotAg0VltgFltCnt) -> MotCtrlMotAg0VltgFltCnt/1
  Process MotAg0 Angle/2(MotCtrlMotAg0ParFltCnt) -> MotCtrlMotAg0ParFltCnt/1
  MotCtrlMotAgMecl0Polarity/1 -> Compensate MechMtrPos1/2(MotCtrlMotAgMecl0Polarity)
  Direct Lookup Table (n-D)2/1 -> Data Store Write2/1, LimDyn_u32/1
  Direct Lookup Table (n-D)1/1 -> Data Store Write1/1, Terminator3/1
  Direct Lookup Table (n-D)/1 -> Data Store Write/1, Process MotAg0 Angle/1(MotAg0Reg_Cnt_u32)
  Process MotAg0 Angle/3(MotCtrlMotAg0MeclRollgCntr) -> MotCtrlMotAg0MeclRollgCntr/1
  Process MotAg0 Angle/4(MotAg0RawMecl) -> Compensate MechMtrPos1/1(MotAg0RawMecl)
  Compensate MechMtrPos1/1(MotAg0Mecl) -> FltInj_u0p16/1(Signal_In)
  FLTINJ_CURRMEAS_MOTCURRCORRDA7/1 -> FltInj_u0p16/2(Constant)
  FltInj_u0p16/1(Signal_Out) -> MotCtrlMotAg0Mecl/1
  FLTINJ_CURRMEAS_MOTCURRCORRDA1/1 -> LimDyn_u32/2
  FLTINJ_CURRMEAS_MOTCURRCORRDA2/1 -> LimDyn_u32/3
  LimDyn_u32/1 -> MotCtrlMotAg0ErrReg/1

== system CM620A_MotAg0Meas/MotAg0Meas/MotAg0MeasPer2 ==
  MotAg0ErrReg : Inport
  MotAg0ParFltCnt : Inport  Port=2
  MotAg0VltgFltCnt : Inport  Port=3
  function : TriggerPort  TriggerType=function-call
  CopyRight2 : Subsystem  Description=|  mask(Copyright Information){none=on}
      | Copyright info block.                                               
      |                                                                     
      | Place copyright information at the top of every subsystem in design.
      mask prompts: none "No parameters"
      mask help: Place copyright information at the top of every subsystem in design.
      mask Display:
      | NxtrConf = 'Nexteer Confidential';
      | 
      | sys = bdroot; %handle for the current model ("system")
      | first = get_param(sys,'Created');
      | first = first(end-3:end);  %year is last four digits
      | 
      | last = get_param(sys,'LastModifiedDate');
      | if isempty(last)
      |     last = datestr(now,'yyyy');
      | else
      |     last = last(end-3:end);
      | end
      | 
      | if strcmp(first,last)
      |     fprintf('%s -- Copyright %s Nexteer',NxtrConf,first)
      | else
      |     fprintf('%s -- %s%s- %s Nexteer',NxtrConf,char(169),first,last)
      | end
  MotAg0 Protocol Fault Operation : Subsystem  RequirementInfo={'linktype_rmi_doors' '0000c47b (/ESG Group/FDD Module Requirements/EA4 Specific/CM620A_MotAg0Meas)' '#CM620A_25' 'true' 'REQ: CM620A_25' '' } %GIDa_7fd546fd_48e1_4d9b_848f_bb77aa877077
  Process ErrorReg and DieRevCtr : Subsystem
  MotAg0Qlfr : Outport  RequirementInfo={} %GIDa_3fc77e2f_6462_49ba_96ea_6336984b6724
  wires:
  MotAg0ErrReg/1 -> Process ErrorReg and DieRevCtr/1(MotAg0ErrReg)
  Process ErrorReg and DieRevCtr/1(MotAg0Err) -> MotAg0 Protocol Fault Operation/1(MotAg0Err)
  Process ErrorReg and DieRevCtr/2(MotAg0ErrParFltCnt) -> MotAg0 Protocol Fault Operation/2(MotAg0ErrParFltCnt)
  MotAg0 Protocol Fault Operation/1(MotAg0Qlfr) -> MotAg0Qlfr/1
  MotAg0ParFltCnt/1 -> MotAg0 Protocol Fault Operation/3(MotAg0ParFltCnt)
  MotAg0VltgFltCnt/1 -> MotAg0 Protocol Fault Operation/4(MotAg0VltgFltCnt)

== system CM620A_MotAg0Meas/Signal Creation/CopyRight2 ==

== system CM620A_MotAg0Meas/MotAg0Meas/MotAg0MeasInit1/Compute Correction Table ==
  CopyRight2 : Subsystem  Description=|  mask(Copyright Information){none=on}
      | Copyright info block.                                               
      |                                                                     
      | Place copyright information at the top of every subsystem in design.
      mask prompts: none "No parameters"
      mask help: Place copyright information at the top of every subsystem in design.
      mask Display:
      | NxtrConf = 'Nexteer Confidential';
      | 
      | sys = bdroot; %handle for the current model ("system")
      | first = get_param(sys,'Created');
      | first = first(end-3:end);  %year is last four digits
      | 
      | last = get_param(sys,'LastModifiedDate');
      | if isempty(last)
      |     last = datestr(now,'yyyy');
      | else
      |     last = last(end-3:end);
      | end
      | 
      | if strcmp(first,last)
      |     fprintf('%s -- Copyright %s Nexteer',NxtrConf,first)
      | else
      |     fprintf('%s -- %s%s- %s Nexteer',NxtrConf,char(169),first,last)
      | end
  If : If  IfExpression=u1 == 0
  MotAg0CoeffTbl_GetErrorStatus : Subsystem  TreatAsAtomicUnit=on
  NVM NOK : Subsystem  TreatAsAtomicUnit=on
  NVM Ok : Subsystem  TreatAsAtomicUnit=on
  wires:
  MotAg0CoeffTbl_GetErrorStatus/1(RequestResultPtr) -> If/1
  If/1 -> NVM Ok/Action
  If/2 -> NVM NOK/Action

== system CM620A_MotAg0Meas/MotAg0Meas/MotAg0MeasInit1/CopyRight2 ==

== system CM620A_MotAg0Meas/MotAg0Meas/MotAg0MeasInit1/Initialize CSIH Registers ==
  note: 1.  Configure the CSIH1 registers according to CM620A_MotAg0Meas_RegisterConfiguration.xlsm
      |     Order by Row.
  CopyRight2 : Subsystem  Description=|  mask(Copyright Information){none=on}
      | Copyright info block.                                               
      |                                                                     
      | Place copyright information at the top of every subsystem in design.
      mask prompts: none "No parameters"
      mask help: Place copyright information at the top of every subsystem in design.
      mask Display:
      | NxtrConf = 'Nexteer Confidential';
      | 
      | sys = bdroot; %handle for the current model ("system")
      | first = get_param(sys,'Created');
      | first = first(end-3:end);  %year is last four digits
      | 
      | last = get_param(sys,'LastModifiedDate');
      | if isempty(last)
      |     last = datestr(now,'yyyy');
      | else
      |     last = last(end-3:end);
      | end
      | 
      | if strcmp(first,last)
      |     fprintf('%s -- Copyright %s Nexteer',NxtrConf,first)
      | else
      |     fprintf('%s -- %s%s- %s Nexteer',NxtrConf,char(169),first,last)
      | end

== system CM620A_MotAg0Meas/MotAg0Meas/MotAg0MeasMotAg0CoeffTblRead/Copyright1 ==

== system CM620A_MotAg0Meas/MotAg0Meas/MotAg0MeasMotAg0CoeffTblWr/Copyright1 ==

== system CM620A_MotAg0Meas/MotAg0Meas/MotAg0MeasMotAg0CoeffTblWr/MotAg0CoeffTbl_SetRamBlockStatus ==
  note: This is the block representing the client call
  BlockChanged : Inport
  Terminator : Terminator
  wires:
  BlockChanged/1 -> Terminator/1

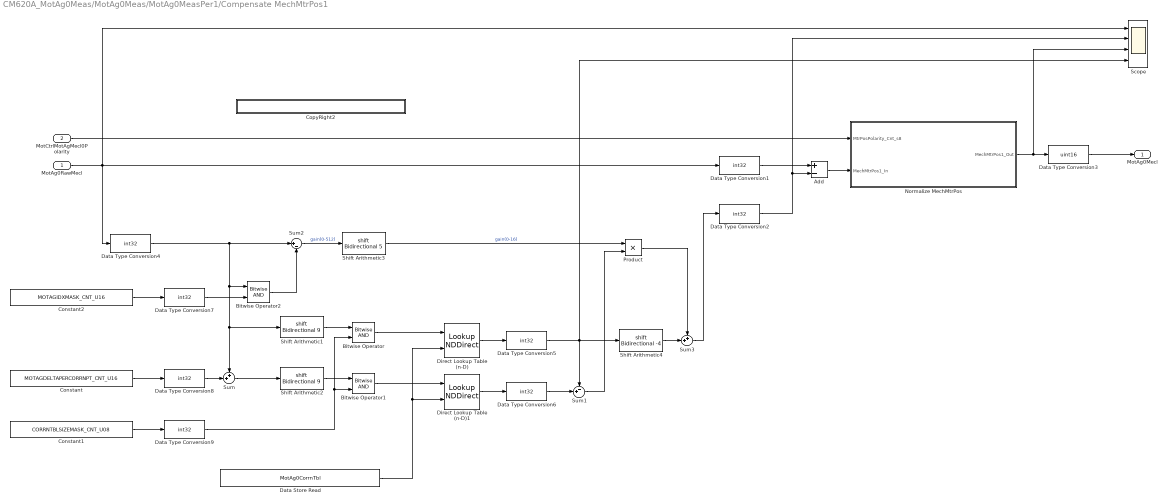
== system CM620A_MotAg0Meas/MotAg0Meas/MotAg0MeasPer1/Compensate MechMtrPos1 ==
  MotAg0RawMecl : Inport
  MotCtrlMotAgMecl0Polarity : Inport  Port=2
  Add : Sum  RequirementInfo={'linktype_rmi_doors' '0000c47b (/ESG Group/FDD Module Requirements/EA4 Specific/CM620A_MotAg0Meas)' '#CM620A_89' 'true' 'REQ: CM620A_89' '' } %GIDa_19103b05_48c4_4017_a459_e28f509a6931  Inputs=+-
  Bitwise Operator : simulink/Logic and Bit Operations/Bitwise Operator  logicop=AND  UseBitMask=off  NumInputPorts=2  BitMask=CORRNTBLSIZEMASK_CNT_U08  BitMaskRealWorld=Stored Integer
  Bitwise Operator1 : simulink/Logic and Bit Operations/Bitwise Operator  logicop=AND  UseBitMask=off  NumInputPorts=2  BitMask=CORRNTBLSIZEMASK_CNT_U08  BitMaskRealWorld=Stored Integer
  Bitwise Operator2 : simulink/Logic and Bit Operations/Bitwise Operator  logicop=AND  UseBitMask=off  NumInputPorts=2  BitMask=MOTAGIDXMASK_CNT_U16  BitMaskRealWorld=Stored Integer
  Constant : Constant  Value=MOTAGDELTAPERCORRNPT_CNT_U16
  Constant1 : Constant  Value=CORRNTBLSIZEMASK_CNT_U08
  Constant2 : Constant  Value=MOTAGIDXMASK_CNT_U16
  CopyRight2 : Subsystem  Description=|  mask(Copyright Information){none=on}
      | Copyright info block.                                               
      |                                                                     
      | Place copyright information at the top of every subsystem in design.
      mask prompts: none "No parameters"
      mask help: Place copyright information at the top of every subsystem in design.
      mask Display:
      | NxtrConf = 'Nexteer Confidential';
      | 
      | sys = bdroot; %handle for the current model ("system")
      | first = get_param(sys,'Created');
      | first = first(end-3:end);  %year is last four digits
      | 
      | last = get_param(sys,'LastModifiedDate');
      | if isempty(last)
      |     last = datestr(now,'yyyy');
      | else
      |     last = last(end-3:end);
      | end
      | 
      | if strcmp(first,last)
      |     fprintf('%s -- Copyright %s Nexteer',NxtrConf,first)
      | else
      |     fprintf('%s -- %s%s- %s Nexteer',NxtrConf,char(169),first,last)
      | end
  Data Store Read : DataStoreRead  DataStoreName=MotAg0CorrnTbl
  Data Type Conversion{1..2,4..9} (8 alike) : DataTypeConversion  OutDataTypeStr=int32
  Data Type Conversion3 : DataTypeConversion  OutDataTypeStr=uint16
  Direct Lookup Table (n-D) : LookupNDDirect  NumberOfTableDimensions=1  TableIsInput=on
  Direct Lookup Table (n-D)1 : LookupNDDirect  NumberOfTableDimensions=1  TableIsInput=on
  Normalize MechMtrPos : Stateflow chart  RequirementInfo={'linktype_rmi_doors' '0000c47b (/ESG Group/FDD Module Requirements/EA4 Specific/CM620A_MotAg0Meas)' '#CM620A_90' 'true' 'REQ: CM620A_90' '' } %GIDa_8be31d7e_ea38_46da_8b91_75c6418a33d0  TreatAsAtomicUnit=on
  Product : Product
  Scope : Scope  NumInputPorts=4
      settings: YMin=-5~-5~-5~-5  YMax=5~5~5~5
  Shift Arithmetic1 : ArithShift  BitShiftNumber=9
  Shift Arithmetic2 : ArithShift  BitShiftNumber=9
  Shift Arithmetic3 : ArithShift  BitShiftNumber=5
  Shift Arithmetic4 : ArithShift  BitShiftNumber=-4
  Sum : Sum  Inputs=++|
  Sum1 : Sum  Inputs=-+|
  Sum2 : Sum  Inputs=|+-
  Sum3 : Sum  Inputs=++|
  MotAg0Mecl : Outport
  wires:
  Normalize MechMtrPos/1(MechMtrPos1_Out) -> Scope/3, Data Type Conversion3/1
  MotCtrlMotAgMecl0Polarity/1 -> Normalize MechMtrPos/1(MtrPosPolarity_Cnt_s8)
  Add/1 -> Normalize MechMtrPos/2(MechMtrPos1_In)
  Shift Arithmetic1/1 -> Bitwise Operator/1
  Data Type Conversion1/1 -> Add/1
  Data Type Conversion2/1 -> Scope/2, Add/2
  Data Type Conversion3/1 -> MotAg0Mecl/1
  MotAg0RawMecl/1 -> Scope/1, Data Type Conversion1/1, Data Type Conversion4/1
  Data Type Conversion4/1 -> Sum/1, Shift Arithmetic1/1, Bitwise Operator2/1, Sum2/1
  Constant/1 -> Data Type Conversion8/1
  Sum/1 -> Shift Arithmetic2/1
  Bitwise Operator/1 -> Direct Lookup Table (n-D)/1
  Shift Arithmetic2/1 -> Bitwise Operator1/1
  Bitwise Operator1/1 -> Direct Lookup Table (n-D)1/1
  Data Store Read/1 -> Direct Lookup Table (n-D)/2, Direct Lookup Table (n-D)1/2
  Direct Lookup Table (n-D)/1 -> Data Type Conversion5/1
  Direct Lookup Table (n-D)1/1 -> Data Type Conversion6/1
  Data Type Conversion5/1 -> Scope/4, Shift Arithmetic4/1, Sum1/1
  Data Type Conversion6/1 -> Sum1/2
  Bitwise Operator2/1 -> Sum2/2
  Sum2/1 -> Shift Arithmetic3/1  "gain(0-512)"
  Shift Arithmetic3/1 -> Product/1  "gain(0-16)"
  Sum1/1 -> Product/2
  Product/1 -> Sum3/1
  Shift Arithmetic4/1 -> Sum3/2
  Sum3/1 -> Data Type Conversion2/1
  Constant1/1 -> Data Type Conversion9/1
  Constant2/1 -> Data Type Conversion7/1
  Data Type Conversion7/1 -> Bitwise Operator2/2
  Data Type Conversion8/1 -> Sum/2
  Data Type Conversion9/1 -> Bitwise Operator1/2, Bitwise Operator/2

== system CM620A_MotAg0Meas/MotAg0Meas/MotAg0MeasPer1/CopyRight2 ==

== system CM620A_MotAg0Meas/MotAg0Meas/MotAg0MeasPer1/FltInj_u0p16 ==
  note: This block requires no modification by FDD author.
      |
      | This block does not actually simulate any fault injection.  It is simply a pass-thru.
      |
      | The Constant port (#2) simply terminates its signal, but we are trying to force the FDD author
      | to properly use the FltInjectionLocType enumeration in FDD model.
  note: EA4.x Fault Injection
  Signal_In : Inport
  Constant : Inport  Port=2
  Copyright1 : Subsystem  Description=|  RequirementInfo={} %GIDa_87d37d2f_bb6d_41e7_bb47_cf6d41a215eb  mask(Copyright Information){none=on}
      | Copyright info block.                                               
      |                                                                     
      | Place copyright information at the top of every subsystem in design.
      mask prompts: none "No parameters"
      mask help: Place copyright information at the top of every subsystem in design.
      mask Display:
      | NxtrConf = 'Nexteer Confidential';
      | 
      | sys = bdroot; %handle for the current model ("system")
      | first = get_param(sys,'Created');
      | if(isempty(first))
      |     first = datestr(now,'yyyy');
      | else
      |     first = first(end-3:end);  %year is last four digits
      | end
      | 
      | last = get_param(sys,'LastModifiedDate');
      | if isempty(last)
      |     last = datestr(now,'yyyy');
      | else
      |     last = last(end-3:end);
      | end
      | 
      | if strcmp(first,last)
      |     fprintf('%s\nCopyright  %s Nexteer',NxtrConf,first);
      | else
      |     fprintf('%s\n%s%s-%s Nexteer',NxtrConf,char(169),first,last);
      | end
  Terminator : Terminator
  Signal_Out : Outport
  wires:
  Signal_In/1 -> Signal_Out/1
  Constant/1 -> Terminator/1

== system CM620A_MotAg0Meas/MotAg0Meas/MotAg0MeasPer1/GetRefTmr1MicroSec32bit ==
  note: Dont code, simulation purposes only
  CopyRight2 : Subsystem  Description=|  mask(Copyright Information){none=on}
      | Copyright info block.                                               
      |                                                                     
      | Place copyright information at the top of every subsystem in design.
      mask prompts: none "No parameters"
      mask help: Place copyright information at the top of every subsystem in design.
      mask Display:
      | NxtrConf = 'Nexteer Confidential';
      | 
      | sys = bdroot; %handle for the current model ("system")
      | first = get_param(sys,'Created');
      | first = first(end-3:end);  %year is last four digits
      | 
      | last = get_param(sys,'LastModifiedDate');
      | if isempty(last)
      |     last = datestr(now,'yyyy');
      | else
      |     last = last(end-3:end);
      | end
      | 
      | if strcmp(first,last)
      |     fprintf('%s -- Copyright %s Nexteer',NxtrConf,first)
      | else
      |     fprintf('%s -- %s%s- %s Nexteer',NxtrConf,char(169),first,last)
      | end
  Data Type Conversion : DataTypeConversion  OutDataTypeStr=uint32
  Gain : Gain  Gain=1000000
  SystemTime : DigitalClock  RequirementInfo={} %GIDa_de5f53aa_11f9_4923_a9e9_0d2d8daf0a33  SampleTime=-1
  RefTmr : Outport
  wires:
  SystemTime/1 -> Gain/1
  Gain/1 -> Data Type Conversion/1
  Data Type Conversion/1 -> RefTmr/1
